simulink model "GridS"  (R2022a)
settings: Solver=FixedStepDiscrete  StartTime=0.0  StopTime=5  RelTol=1e-3
values from neighbouring files (symbols this model uses):
  Clink = Ceq*2    (= 0.217013888889)    [Set_parameters_R2018.m]
  Fc = 33 * Fnom    (= 1980)    [Set_parameters_R2018.m]
  Fnom = 60    [Set_parameters_R2018.m]
  Increment_MPPT = 0.01    [Set_parameters_R2018.m]
  Ki_Ireg = 20    [Set_parameters_R2018.m]
  Ki_VDCreg = 400    [Set_parameters_R2018.m]
  Kp_Ireg = 0.3    [Set_parameters_R2018.m]
  Kp_VDCreg = 2    [Set_parameters_R2018.m]
  LimitL_Ireg = -1.5    [Set_parameters_R2018.m]
  LimitL_VDCreg = -1.5    [Set_parameters_R2018.m]
  Limits_MPPT = [ 583 357 ]    [Set_parameters_R2018.m]
  LimitU_Ireg = 1.5    [Set_parameters_R2018.m]
  LimitU_VDCreg = 1.5    [Set_parameters_R2018.m]
  Pnom = 1e6    (= 1000000)    [Set_parameters_R2018.m]
  Ts_Control = 10*Ts_Power    (= 5.05050505051e-05)    [Set_parameters_R2018.m]
  Ts_Power = 1/(33*Fnom)/100    (= 5.05050505051e-06)    [Set_parameters_R2018.m]
  Vf = 0    [Set_parameters_R2018.m]
  Vfd = 0    [Set_parameters_R2018.m]
  Vnom_dc = 480    [Set_parameters_R2018.m]
  Vnom_Diesel = 2.4e3    (= 2400)    [Set_parameters_R2018.m]
  Vnom_prim = 13.8e3    (= 13800)    [Set_parameters_R2018.m]
  Vnom_sec = 220    [Set_parameters_R2018.m]
undefined symbols (not defined in the file or in its folder): D1, Delta, RL, RLff, sigbuilder_block
libraries: spsLoadFlowBusLib x7, spsThreePhasePISectionLineLib x6, spsThreePhaseSeriesRLCLoadLib x4, spsThreePhaseTransformerTwoWindingsLib x3, spsThreePhaseBreakerLib x2, spsThreePhaseVIMeasurementLib x2, spsThreePhaseSeriesRLCBranchLib x2, spsSeriesRLCBranchLib x2, slpidlib x2, spsabctodq0Lib x2, spsVoltageMeasurementLib x2, spsPVArrayLib x1
settings Model: Creator=z0034ktr  LastModifiedBy=pdutt
settings SolverCC: AlgebraicLoopSolver=TrustRegion
settings DebuggingCC: IgnoredZcDiagnostic=none  UnconnectedInputMsg=warning  UnconnectedOutputMsg=warning  UnconnectedLineMsg=warning  SFMachineParentedDataDiag=warning

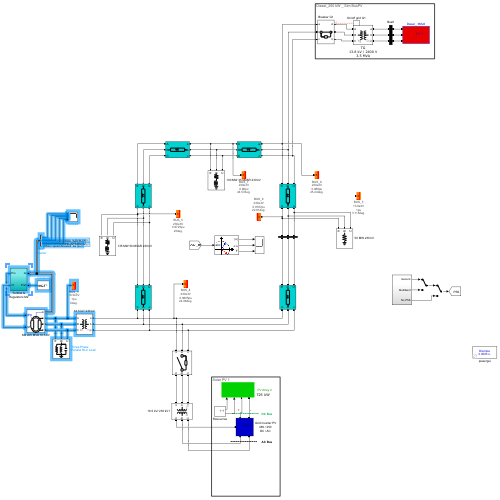
[thumbnail: Simulink's stored preview of the top-level diagram]
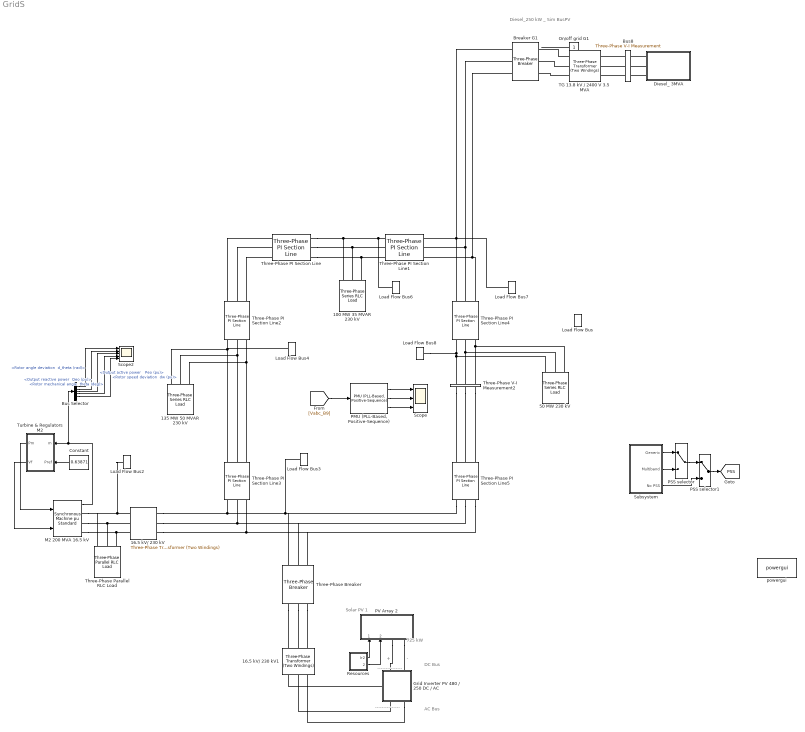
== system GridS ==
  note: -
  note: +
  note: ---------------
  note: ---------------
  note: Solar PV 1
  note: 725 kW
  note: DC Bus
  note: AC Bus
  note: Diesel_250 kW _ Sim BusPV
  "  PV Array 2" : Subsystem
      mask Display: image(imread('Icons\PV.png'));
  100 MW 35 MVAR 230 kV : spsThreePhaseSeriesRLCLoadLib/Three-Phase Series RLC Load  LConnTagsString=A|B|C  Configuration=Y (grounded)  NominalVoltage=(230000)*0.980041  Vabc=[1e3 1e3 1e3]  Vabcp=[1e3 1e3 1e3]  NominalFrequency=60  UnbalancedPower=off  ActivePower=100e6  InductivePower=35e6  CapacitivePower=0  Pabc=[10e3 9e3 11e3]  QLabc=[100 90 110]  QCabc=[100 90 110]  Pabcp=[10e3 9e3 11e3]  QLabcp=[100 90 110]  QCabcp=[100 90 110]  Measurements=None  LoadType=constant PQ
  135 MW 50 MVAR 230 kV : spsThreePhaseSeriesRLCLoadLib/Three-Phase Series RLC Load  LConnTagsString=A|B|C  Configuration=Y (grounded)  NominalVoltage=(230000)*0.972469  Vabc=[1e3 1e3 1e3]  Vabcp=[1e3 1e3 1e3]  NominalFrequency=60  UnbalancedPower=off  ActivePower=135e6  InductivePower=50e6  CapacitivePower=0  Pabc=[10e3 9e3 11e3]  QLabc=[100 90 110]  QCabc=[100 90 110]  Pabcp=[10e3 9e3 11e3]  QLabcp=[100 90 110]  QCabcp=[100 90 110]  Measurements=None  LoadType=constant PQ
  16.5 kV/ 230 kV : spsThreePhaseTransformerTwoWindingsLib/Three-Phase Transformer (Two Windings)  Winding1Connection=Delta (D1)  Winding2Connection=Yg  CoreType=Three single-phase transformers  SetSaturation=off  Hysteresis=off  DataFile='hysteresis'  SetInitialFlux=off  Measurements=None  UNITS=pu  NominalPower=[ 200e6 , 60 ]  Winding1=[ 16.5e3 , 0.002 , 0.08 ]  Winding2=[ 230e3 , 0.002 , 0.08 ]  Rm=500  Lm=500  L0=0.5  Saturation=[ 0,0 ; 0.0024,1.2 ; 1.0,1.52 ]  InitialFluxes=[ 0.8 , -0.8 , 0.7 ]  BreakLoop=off  DiscreteSolver=Trapezoidal iterative  DataType=off  TransfoNumber=1
  16.5 kV/ 230 kV1 : spsThreePhaseTransformerTwoWindingsLib/Three-Phase Transformer (Two Windings)  Winding1Connection=Delta (D1)  Winding2Connection=Yg  CoreType=Three single-phase transformers  SetSaturation=off  Hysteresis=off  DataFile='hysteresis'  SetInitialFlux=off  Measurements=None  UNITS=pu  NominalPower=[ 200e6 , 60 ]  Winding1=[ 250 , 0.002 , 0.08 ]  Winding2=[ 230e3 , 0.002 , 0.08 ]  Rm=500  Lm=500  L0=0.5  Saturation=[ 0,0 ; 0.0024,1.2 ; 1.0,1.52 ]  InitialFluxes=[ 0.8 , -0.8 , 0.7 ]  BreakLoop=off  DiscreteSolver=Trapezoidal iterative  DataType=off  TransfoNumber=1
  50 MW 230 kV : spsThreePhaseSeriesRLCLoadLib/Three-Phase Series RLC Load  LConnTagsString=A|B|C  Configuration=Y (grounded)  NominalVoltage=(230000)*0.978663  Vabc=[1e3 1e3 1e3]  Vabcp=[1e3 1e3 1e3]  NominalFrequency=60  UnbalancedPower=off  ActivePower=50e6  InductivePower=0  CapacitivePower=0  Pabc=[10e3 9e3 11e3]  QLabc=[100 90 110]  QCabc=[100 90 110]  Pabcp=[10e3 9e3 11e3]  QLabcp=[100 90 110]  QCabcp=[100 90 110]  Measurements=None  LoadType=constant PQ
  Breaker G1 : spsThreePhaseBreakerLib/Three-Phase Breaker  InitialState=closed  SwitchA=on  SwitchB=on  SwitchC=on  SwitchTimes=[3 5]  External=off  BreakerResistance=0.001  SnubberResistance=1e6  SnubberCapacitance=inf  Measurements=None
  Bus Selector : BusSelector  OutputSignals="Mechanical.Rotor angle deviation  d_theta (rad),Output reactive power  Qeo (pu),Output active power   Peo (pu),Mechanical.Rotor mechanical angle  theta (deg),Mechanical.Rotor speed deviation  dw (pu)"
  Bus8 : spsThreePhaseVIMeasurementLib/Three-Phase V-I Measurement  VoltageMeasurement=phase-to-ground  SetLabelV=on  LabelV=VabcLL_Bus_8  Vpu=off  VpuLL=off  CurrentMeasurement=yes  SetLabelI=on  LabelI=IabcLL_Bus_8  Ipu=off  Pbase=100e6  Vbase=25e3/sqrt(2)  OutputType=Complex  PhasorSimulation=off  PSBequivalent=0
  Constant : Constant  Value=0.63871
  Diesel_ 3MVA : Subsystem
      mask Display: image(imread('Icons\Diesel 50kW1.png'));
  "Grid Inverter PV 480 / 250 DC / AC " : Subsystem
      settings: PortSchema="{\"entries\":[{\"content\":{\"sides\":[{\"content\":{\"connectorIds\":[\"LConn1\",\"LConn2\"]},\"type\":\"ConnectorPlacement.EquallySpacedRectSide\",\"uuid\":\"ac79584a-c7d0-4a74-aa4d-67aed92924e2\"},{\"content\":{\"connectorIds\":[\"RConn1\",\"RConn2\"],\"side\":\"RIGHT\"},\"type\":\"ConnectorPlacement.EquallySpacedRectSide\",\"uuid\":\"44d96f25-a8f9-47e8-b296-82c7ffbfe922\"},{\"content\":{\"connectorIds\":[\"LConn3\"],\"side\":\"TOP\"},\"type\":\"ConnectorPlacement.EquallySpacedRectSide\",\"uuid\":\"f35e0256-66c3-4b52-94e0-36412c815474\"}]},\"type\":\"ConnectorPlacement.EquallySpacedConnector\",\"uuid\":\"6af4db4f-53ba-4d1f-a030-0edda350e303\"}],\"packageUris\":[\"http://schema.mathworks.com/mf0/Connector/R2020b\"],\"version\":\"1.0\"}"
      mask Display: image(imread('Icons\Inverter.png'));
  Load Flow Bus : spsLoadFlowBusLib/Load Flow Bus  LConnTagsString=a  Phases=single  Connectors=on one side  ID=BUS_3  Vbase=13.8e3  Vref=1  Vangle=0  VLF=1  VLFb=1  VLFc=1  angleLF=3.115  angleLFb=0  angleLFc=0
      settings: SourceProductBaseCode=PS
  Load Flow Bus2 : spsLoadFlowBusLib/Load Flow Bus  LConnTagsString=a  Phases=single  Connectors=on one side  ID=BUS_1  Vbase=16.5e3  Vref=1  Vangle=0  VLF=1  VLFb=1  VLFc=1  angleLF=0  angleLFb=0  angleLFc=0
      settings: SourceProductBaseCode=PS
  Load Flow Bus3 : spsLoadFlowBusLib/Load Flow Bus  LConnTagsString=a  Phases=single  Connectors=on one side  ID=BUS_4  Vbase=230e3  Vref=1  Vangle=0  VLF=0.9805  VLFb=1  VLFc=1  angleLF=24.06  angleLFb=0  angleLFc=0
      settings: SourceProductBaseCode=PS
  Load Flow Bus4 : spsLoadFlowBusLib/Load Flow Bus  LConnTagsString=a  Phases=single  Connectors=on one side  ID=BUS_5  Vbase=230e3  Vref=1  Vangle=0  VLF=0.9725  VLFb=1  VLFc=1  angleLF=23  angleLFb=0  angleLFc=0
      settings: SourceProductBaseCode=PS
  Load Flow Bus6 : spsLoadFlowBusLib/Load Flow Bus  LConnTagsString=a  Phases=single  Connectors=on one side  ID=BUS_7  Vbase=230e3  Vref=1  Vangle=0  VLF=0.98  VLFb=1  VLFc=1  angleLF=24.57  angleLFb=0  angleLFc=0
      settings: SourceProductBaseCode=PS
  Load Flow Bus7 : spsLoadFlowBusLib/Load Flow Bus  LConnTagsString=a  Phases=single  Connectors=on one side  ID=BUS_8  Vbase=230e3  Vref=1  Vangle=0  VLF=0.988  VLFb=1  VLFc=1  angleLF=25.24  angleLFb=0  angleLFc=0
      settings: SourceProductBaseCode=PS
  Load Flow Bus8 : spsLoadFlowBusLib/Load Flow Bus  LConnTagsString=a  Phases=single  Connectors=on one side  ID=BUS_9  Vbase=230e3  Vref=1  Vangle=0  VLF=0.9787  VLFb=1  VLFc=1  angleLF=22.61  angleLFb=0  angleLFc=0
      settings: SourceProductBaseCode=PS
  M2 200 MVA 16.5 kV : spsSynchronousMachinepuStandardLib/Synchronous Machine pu Standard  PresetModel=No  MechanicalLoad=Mechanical power Pm  ShowDetailedParameters=on  RotorType=Salient-pole  Units=per unit standard parameters  MeasurementBus=off  NominalParameters="[200E6  16500   60 ]"  Reactances1=[ 31 32 33 34 35 36 37 ]  Reactances2=[ 1.305, 0.296, 0.252, 0.474, 0.243, 0.18 ]  dAxisTimeConstants=Short-circuit  qAxisTimeConstants=Open-circuit  TimeConstants1=[]  TimeConstants2=[]  TimeConstants3=[]  TimeConstants4=[]  TimeConstants5=[ 1.01, 0.053, 0.1 ]  TimeConstants6=[]  TimeConstants7=[]  TimeConstants8=[]  StatorResistance=2.8544e-3  Mechanical="[ 3.7 0  32]"  PolePairs=32  InitialConditions=[0 -74.1936 0.653801 0.653801 0.653801 -12.3345 -132.335 107.665 1.36624]  SetSaturation=off  Saturation=[0.6404,0.7127,0.8441,0.9214,0.9956,1.082,1.19,1.316,1.457;0.7,0.7698,0.8872,0.9466,0.9969,1.046,1.1,1.151,1.201]  LoadFlowParameters=[2 4000000000 0 0]  TsPowergui=0  TsBlock=-1  IterativeModel=Trapezoidal non iterative  IterativeDiscreteModel=Trapezoidal non iterative  BusType=swing  Pref=0  Qref=0  Qmin=-Inf  Qmax=Inf  PLF=0  QLF=0
      settings: SourceProductName=Specialized Power Systems
  On/off grid G1 : Constant
  "PMU (PLL-Based, Positive-Sequence)" : spsPMUPLLBasedPositiveSequenceLib/PMU (PLL-Based, Positive-Sequence)  nominalFrequency=60  samplingRate=64  reportingFactor=1
      settings: SourceProductBaseCode=PS
  PSS selector : ManualSwitch
  PSS selector1 : ManualSwitch
  Resources : Subsystem
      mask Display: image(imread('Icons\R_Sol.jpg'));
  Scope : Scope  NumInputPorts=3
  Scope2 : Scope  NumInputPorts=5
  Subsystem : Subsystem
  TG 13.8 kV / 2400 V 3.5 MVA : spsThreePhaseTransformerTwoWindingsLib/Three-Phase Transformer (Two Windings)  Winding1Connection=Yg  Winding2Connection=Delta (D1)  CoreType=Three single-phase transformers  SetSaturation=off  Hysteresis=off  DataFile='hysteresis'  SetInitialFlux=off  Measurements=None  UNITS=pu  NominalPower=[3.5e6 , Fnom ]  Winding1=[ 230e3, 0.015/2 , 0.015/2/377]  Winding2=[ Vnom_Diesel , 0.015/2 , 0.015/2/377]  Rm=500  Lm=500  L0=0.5  Saturation="[ 0,0  ;  0.005,1.2  ;  1.0,1.4 ]"  InitialFluxes=[ 0.8 , -0.8 , 0.7 ]  BreakLoop=off  DiscreteSolver=Trapezoidal iterative  DataType=off  TransfoNumber=0
  Three-Phase PI Section Line : spsThreePhasePISectionLineLib/Three-Phase PI Section Line  LConnTagsString=a|b|c  RConnTagsString=A|B|C  Length=50  Frequency=60  Resistances=[ 0.01273 0.3864]  Inductances="[ 0.9337e-3  4.1264e-3]"  Capacitances=[12.74e-9 7.751e-9]
  Three-Phase PI Section Line1 : spsThreePhasePISectionLineLib/Three-Phase PI Section Line  LConnTagsString=a|b|c  RConnTagsString=A|B|C  Length=100  Frequency=60  Resistances=[ 0.01273 0.3864]  Inductances="[ 0.9337e-3  4.1264e-3]"  Capacitances=[12.74e-9 7.751e-9]
  Three-Phase PI Section Line2 : spsThreePhasePISectionLineLib/Three-Phase PI Section Line  LConnTagsString=a|b|c  RConnTagsString=A|B|C  Length=100  Frequency=60  Resistances=[ 0.01273 0.3864]  Inductances="[ 0.9337e-3  4.1264e-3]"  Capacitances=[12.74e-9 7.751e-9]
  Three-Phase PI Section Line3 : spsThreePhasePISectionLineLib/Three-Phase PI Section Line  LConnTagsString=a|b|c  RConnTagsString=A|B|C  Length=50  Frequency=60  Resistances=[ 0.01273 0.3864]  Inductances="[ 0.9337e-3  4.1264e-3]"  Capacitances=[12.74e-9 7.751e-9]
  Three-Phase PI Section Line4 : spsThreePhasePISectionLineLib/Three-Phase PI Section Line  LConnTagsString=a|b|c  RConnTagsString=A|B|C  Length=100  Frequency=60  Resistances=[ 0.01273 0.3864]  Inductances="[ 0.9337e-3  4.1264e-3]"  Capacitances=[12.74e-9 7.751e-9]
  Three-Phase PI Section Line5 : spsThreePhasePISectionLineLib/Three-Phase PI Section Line  LConnTagsString=a|b|c  RConnTagsString=A|B|C  Length=50  Frequency=60  Resistances=[ 0.01273 0.3864]  Inductances="[ 0.9337e-3  4.1264e-3]"  Capacitances=[12.74e-9 7.751e-9]
  Three-Phase Parallel RLC Load : spsThreePhaseParallelRLCLoadLib/Three-Phase Parallel RLC Load  LConnTagsString=A|B|C  Configuration=Y (grounded)  NominalVoltage=16.5e3  Vabc=[1e3 1e3 1e3]  Vabcp=[1e3 1e3 1e3]  NominalFrequency=60  UnbalancedPower=off  ActivePower=10e3  InductivePower=100  CapacitivePower=100  Pabc=[10e3 9e3 11e3]  QLabc=[100 90 110]  QCabc=[100 90 110]  Pabcp=[10e3 9e3 11e3]  QLabcp=[100 90 110]  QCabcp=[100 90 110]  Measurements=None  LoadType=constant Z
  Three-Phase V-I Measurement2 : spsThreePhaseVIMeasurementLib/Three-Phase V-I Measurement  VoltageMeasurement=phase-to-phase  SetLabelV=on  LabelV=Vabc_B9  Vpu=off  VpuLL=on  CurrentMeasurement=no  SetLabelI=off  LabelI=Iabc  Ipu=off  Pbase=100e6  Vbase=230e3  OutputType=Complex  PhasorSimulation=off  PSBequivalent=0
  Three-Phase Breaker : spsThreePhaseBreakerLib/Three-Phase Breaker  InitialState=open  SwitchA=on  SwitchB=on  SwitchC=on  SwitchTimes=[2 5]  External=off  BreakerResistance=0.01  SnubberResistance=1e6  SnubberCapacitance=inf  Measurements=None
  Turbine & Regulators M2 : Subsystem
  powergui : spspowerguiLib/powergui  Priority=1  SimulationMode=Discrete  SampleTime=50e-5  frequency=60  Iterations=50  frequencyindice=60  Pbase=200  ErrMax=0.0001  UnitsV=kV  UnitsW=MW  buscounter=0  FunctionMessages=off  echomessages=off  EnableUseOfTLC=off  CurrentSourceSwitches=off  DisableSnubberDevices=off  DisableRonSwitches=off  DisableVfSwitches=off  DisplayEquations=off  AutomaticDiscreteSolvers=off  SolverType=Backward Euler  Interpol=off  ExternalGateDelay=off  methode=off  Ts=100  x0status=blocks  SPID=on  SwTol=0  HookPort=off  NonlinearTolerance=1e-4  nMaxIteration=100  ContinueOnMaxIteration=off  RestoreLinks=warning  ResistiveCurrentMeasurement=off  Frange=[0:2:500]  Ylog=off  Xlog=on  ShowGrid=off  save=off  variable=ZData  structure=0  ZoomFFT=off  StartTime=0.0  cycles=1  DisplayStyle=1  fundamental=60  FreqAxis=off  MaxFrequency=1000  frequencyindicesteady=1  RmsSteady=1  display=off
  tag scope: PSS=global
  wires:
  [Vabc_B9] -> "PMU (PLL-Based, Positive-Sequence)"/1
  "PMU (PLL-Based, Positive-Sequence)"/3 -> Scope/3
  "PMU (PLL-Based, Positive-Sequence)"/2 -> Scope/2
  "PMU (PLL-Based, Positive-Sequence)"/1 -> Scope/1
  M2 200 MVA 16.5 kV/1 -> Bus Selector/1, Turbine & Regulators M2/1(m)
  Turbine & Regulators M2/2(Vf) -> M2 200 MVA 16.5 kV/2
  Turbine & Regulators M2/1(Pm) -> M2 200 MVA 16.5 kV/1
  Constant/1 -> Turbine & Regulators M2/2(Pref)
  PSS selector/1 -> PSS selector1/1
  Subsystem/1(Generic) -> PSS selector/1
  Subsystem/3(No PSS) -> PSS selector1/2
  Subsystem/2(Multiband) -> PSS selector/2
  PSS selector1/1 -> [PSS]
  Bus Selector/1 -> Scope2/1  "<Rotor angle deviation  d_theta (rad)>"
  Bus Selector/2 -> Scope2/2  "<Output reactive power  Qeo (pu)>"
  Bus Selector/3 -> Scope2/3  "<Output active power   Peo (pu)>"
  Bus Selector/4 -> Scope2/4  "<Rotor mechanical angle  theta (deg)>"
  Bus Selector/5 -> Scope2/5  "<Rotor speed deviation  dw (pu)>"
  Resources/1(Ir2) -> "  PV Array 2"/1(Irradiance)
  Resources/2(temp) -> "  PV Array 2"/2(Temp2)
  On/off grid G1/1 -> ?
  connections:
  16.5 kV/ 230 kV/RConn1 -- Three-Phase Breaker/RConn1 -- Three-Phase PI Section Line5/RConn1 -- Load Flow Bus3/LConn1 -- Three-Phase PI Section Line3/RConn1
  16.5 kV/ 230 kV/RConn2 -- Three-Phase Breaker/RConn2 -- Three-Phase PI Section Line5/RConn2 -- Three-Phase PI Section Line3/RConn2
  16.5 kV/ 230 kV/RConn3 -- Three-Phase Breaker/RConn3 -- Three-Phase PI Section Line5/RConn3 -- Three-Phase PI Section Line3/RConn3
  50 MW 230 kV/LConn1 -- Three-Phase PI Section Line4/RConn1 -- Load Flow Bus8/LConn1 -- Three-Phase V-I Measurement2/RConn1
  Three-Phase V-I Measurement2/LConn3 -- Three-Phase PI Section Line5/LConn3
  Three-Phase PI Section Line4/LConn1 -- Breaker G1/RConn1 -- Load Flow Bus7/LConn1 -- Three-Phase PI Section Line1/RConn1
  Three-Phase PI Section Line4/LConn2 -- Breaker G1/RConn2 -- Three-Phase PI Section Line1/RConn2
  Three-Phase PI Section Line4/LConn3 -- Breaker G1/RConn3 -- Three-Phase PI Section Line1/RConn3
  Three-Phase PI Section Line/RConn1 -- 100 MW 35 MVAR 230 kV/LConn1 -- Load Flow Bus6/LConn1 -- Three-Phase PI Section Line1/LConn1
  Three-Phase PI Section Line/RConn2 -- 100 MW 35 MVAR 230 kV/LConn2 -- Three-Phase PI Section Line1/LConn2
  Three-Phase PI Section Line/RConn3 -- 100 MW 35 MVAR 230 kV/LConn3 -- Three-Phase PI Section Line1/LConn3
  Three-Phase PI Section Line3/LConn1 -- Load Flow Bus4/LConn1 -- Three-Phase PI Section Line2/RConn1 -- 135 MW 50 MVAR 230 kV/LConn1
  Three-Phase PI Section Line3/LConn2 -- 135 MW 50 MVAR 230 kV/LConn2 -- Three-Phase PI Section Line2/RConn2
  Three-Phase PI Section Line3/LConn3 -- 135 MW 50 MVAR 230 kV/LConn3 -- Three-Phase PI Section Line2/RConn3
  Three-Phase PI Section Line2/LConn3 -- Three-Phase PI Section Line/LConn3
  Three-Phase PI Section Line2/LConn2 -- Three-Phase PI Section Line/LConn2
  Three-Phase PI Section Line2/LConn1 -- Three-Phase PI Section Line/LConn1
  Load Flow Bus2/LConn1 -- Three-Phase Parallel RLC Load/LConn1 -- M2 200 MVA 16.5 kV/RConn1 -- 16.5 kV/ 230 kV/LConn1
  M2 200 MVA 16.5 kV/RConn2 -- 16.5 kV/ 230 kV/LConn2 -- Three-Phase Parallel RLC Load/LConn2
  M2 200 MVA 16.5 kV/RConn3 -- 16.5 kV/ 230 kV/LConn3 -- Three-Phase Parallel RLC Load/LConn3
  50 MW 230 kV/LConn3 -- Three-Phase V-I Measurement2/RConn3 -- Three-Phase PI Section Line4/RConn3
  Three-Phase V-I Measurement2/LConn2 -- Three-Phase PI Section Line5/LConn2
  Three-Phase V-I Measurement2/LConn1 -- Three-Phase PI Section Line5/LConn1
  50 MW 230 kV/LConn2 -- Three-Phase V-I Measurement2/RConn2 -- Three-Phase PI Section Line4/RConn2
  "  PV Array 2"/LConn1 -- "Grid Inverter PV 480 / 250 DC / AC "/LConn1
  "  PV Array 2"/LConn2 -- "Grid Inverter PV 480 / 250 DC / AC "/LConn2
  "Grid Inverter PV 480 / 250 DC / AC "/LConn3 -- 16.5 kV/ 230 kV1/LConn1
  "Grid Inverter PV 480 / 250 DC / AC "/RConn1 -- 16.5 kV/ 230 kV1/LConn2
  "Grid Inverter PV 480 / 250 DC / AC "/RConn2 -- 16.5 kV/ 230 kV1/LConn3
  Three-Phase Breaker/LConn1 -- 16.5 kV/ 230 kV1/RConn1
  Three-Phase Breaker/LConn2 -- 16.5 kV/ 230 kV1/RConn2
  Three-Phase Breaker/LConn3 -- 16.5 kV/ 230 kV1/RConn3
  Bus8/RConn3 -- TG 13.8 kV / 2400 V 3.5 MVA/RConn3
  Diesel_ 3MVA/LConn1 -- Bus8/LConn1
  Diesel_ 3MVA/LConn2 -- Bus8/LConn2
  TG 13.8 kV / 2400 V 3.5 MVA/LConn2 -- Breaker G1/LConn2
  Bus8/RConn1 -- TG 13.8 kV / 2400 V 3.5 MVA/RConn1
  TG 13.8 kV / 2400 V 3.5 MVA/LConn3 -- Breaker G1/LConn3
  TG 13.8 kV / 2400 V 3.5 MVA/LConn1 -- Breaker G1/LConn1
  Bus8/RConn2 -- TG 13.8 kV / 2400 V 3.5 MVA/RConn2
  Diesel_ 3MVA/LConn3 -- Bus8/LConn3

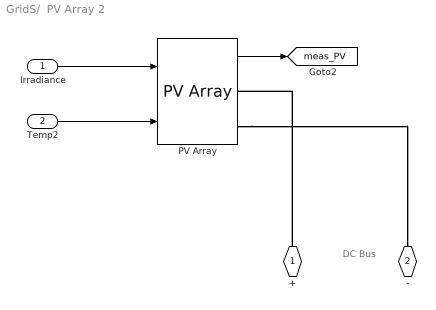
== system GridS/  PV Array 2 ==
  note: DC Bus
  Irradiance : Inport
  Temp2 : Inport  Port=2
  PV Array : spsPVArrayLib/PV Array  Npar=250  Nser=7  PlotType=array @ 1000 W/m2 & specified temperatures  S_vec="[ 1000  500  100 ]"  Temp_C_vec="[ 45 25  ]"  ModuleName=SunPower SPR-415E-WHT-D  PlotWhenSelected=off  Pm=414.801  Ncell=128  Voc=85.3  Isc=6.09  Vm=72.9  Im=5.69  beta_Voc_pc=-0.229  alpha_Isc_pc=0.030706  beta_Voc=-0.19534  alpha_Isc=0.00187  IL=6.0978  I0=7.1698e-13  nI=0.87223  Rsh=419.7781  Rs=0.53711  RobustModel=off  RobustCellTemperature=313.3991  BAL=on  Tc=1e-6  Tfilter=5e-5
      settings: AttributesFormatString=|
      | %<ModuleName>
      | %<Nser>-module string
      | %<Npar> parallel strings
  + : PMIOPort  Tag=PMCPort  Side=Left
  - : PMIOPort  Tag=PMCPort  Port=2  Side=Left
  tag scope: meas_PV=global
  wires:
  PV Array/1 -> [meas_PV]
  Irradiance/1 -> PV Array/1
  Temp2/1 -> PV Array/2
  connections:
  PV Array/RConn2 -- -/RConn1
  +/RConn1 -- PV Array/RConn1

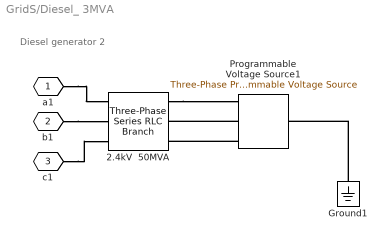
== system GridS/Diesel_ 3MVA ==
  note: Diesel generator 2
  2.4kV  50MVA : spsThreePhaseSeriesRLCBranchLib/Three-Phase Series RLC Branch  LConnTagsString=A|B|C  RConnTagsString=A|B|C  BranchType=RL  Resistance=2.4e3^2/50e6/10  Inductance=2.4e3^2/50e6/(2*pi*60)  Capacitance=1.0  Measurements=None
  Ground1 : spsGroundLib/Ground  LConnTagsString=a
  Programmable Voltage Source1 : spsThreePhaseProgrammableVoltageSourceLib/Three-Phase Programmable Voltage Source  PositiveSequence="[Vnom_Diesel*0.9848 -60  Fnom]"  VariationEntity=None  VariationType=Table of time-amplitude pairs  VariationTypeAlt=Step  VariationStep=-0.3  VariationRate=0.5  VariationMagnitude=0.4  VariationFrequency=2  VariationTiming=[0.1 1.2]  VariationPhaseA=off  Amplitudes=[1]  TimeValues=[0]  HarmonicGeneration=off  HarmonicA=[3 0.2 -25 0]  HarmonicB="[2 0.15  35 2]"  Timing="[0.1  0.6]"  BusType=PV  Pref=Pgen_Diesel  Qref=0  Qmin=-inf  Qmax=inf
  a1 : PMIOPort  Tag=PMCPort  Side=Left
  b1 : PMIOPort  Tag=PMCPort  Port=2  Side=Left
  c1 : PMIOPort  Tag=PMCPort  Port=3  Side=Left
  connections:
  Programmable Voltage Source1/RConn3 -- 2.4kV  50MVA/LConn3
  Ground1/LConn1 -- Programmable Voltage Source1/LConn1
  Programmable Voltage Source1/RConn2 -- 2.4kV  50MVA/LConn2
  2.4kV  50MVA/LConn1 -- Programmable Voltage Source1/RConn1
  b1/RConn1 -- 2.4kV  50MVA/RConn2
  a1/RConn1 -- 2.4kV  50MVA/RConn1
  c1/RConn1 -- 2.4kV  50MVA/RConn3

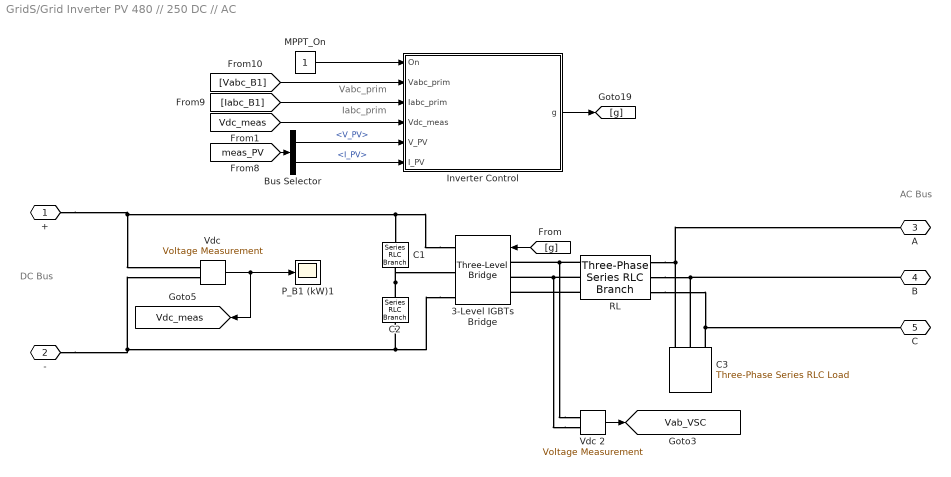
== system GridS/Grid Inverter PV 480 // 250 DC // AC  ==
  note: Iabc_prim
  note: Vabc_prim
  note: AC Bus
  note: DC Bus
  3-Level IGBTs Bridge : spsThreeLevelBridgeLib/Three-Level Bridge  Arms=3  SnubberResistance=Rs  SbubberCapacitance=Cs  Device=IGBT / Diodes  Ron=Ron  ForwardVoltages="[  Vfd  Vf ]"  Measurements=None
      settings: AttributesFormatString=\n  SourceProductBaseCode=PS
  Bus Selector : BusSelector  OutputSignals=V_PV,I_PV
  C1 : spsSeriesRLCBranchLib/Series RLC Branch  LConnTagsString=__new0  RConnTagsString=__new0  BranchType=C  Resistance=1.0  Inductance=1.0  SetiL0=off  InitialCurrent=0  Capacitance=Clink  Setx0=on  InitialVoltage=Vnom_dc/2  Measurements=None
  C2 : spsSeriesRLCBranchLib/Series RLC Branch  LConnTagsString=__new0  RConnTagsString=__new0  BranchType=C  Resistance=1.0  Inductance=1.0  SetiL0=off  InitialCurrent=0  Capacitance=Clink  Setx0=on  InitialVoltage=Vnom_dc/2  Measurements=None
  C3 : spsThreePhaseSeriesRLCLoadLib/Three-Phase Series RLC Load  LConnTagsString=A|B|C  Configuration=Delta  NominalVoltage=Vnom_sec  Vabc=[1e3 1e3 1e3]  Vabcp=[1e3 1e3 1e3]  NominalFrequency=Fnom  UnbalancedPower=off  ActivePower=Pc  InductivePower=0  CapacitivePower=Qc  Pabc=[10e3 9e3 11e3]  QLabc=[100 90 110]  QCabc=[100 90 110]  Pabcp=[10e3 9e3 11e3]  QLabcp=[100 90 110]  QCabcp=[100 90 110]  Measurements=None  LoadType=constant Z
  Inverter Control : Subsystem  mask(Inverter Control){Pnom=Pnom, Fnom=Fnom, Vnom_prim=Vnom_prim, Vnom_sec=Vnom_sec, Vnom_dc=Vnom_dc, Increment_MPPT=Increment_MPPT, Limits_MPPT=Limits_MPPT, Vdc_ref_Init=Vnom_dc, Kp_VDCreg=Kp_VDCreg, Ki_VDCreg=Ki_VDCreg, Kp_Ireg=Kp_Ireg, Ki_Ireg=Ki_Ireg, RLff=RLff, Fc=Fc, Ts_Control=Ts_Control, Ts_PWMgenerator=Ts_Power}
      mask prompts: Pnom "Power (VA)"; Fnom "Frequency (Hz)"; Vnom_prim "Primary voltage (Vrms LL)"; Vnom_sec "Secondary voltage (Vrms LL)"; Vnom_dc "DC voltage (V)"; Increment_MPPT "Output increment (V)"; Limits_MPPT "Output limits [ Upper  Lower ]"; Vdc_ref_Init "Output initial value (V)"; Kp_VDCreg "Proportional gain"; Ki_VDCreg "Integral gain"; Kp_Ireg "Proportional gain"; Ki_Ireg "Integral gain"; RLff "Feedforward Values [Rff Lff]"; Fc "Carrier frequency (Hz)"; Ts_Control "Control systems"; Ts_PWMgenerator "PWM generator"
      mask help:
      | The main components of the Inverter Control are:
      | 1. PLL & Measurements
      | 2. Maximum Power Point Tracker System (MPPT) using a Perturb & Observe algorithm
      | 3. DC Voltage Regulator
      | 4. Current Regulator
      | 5. PWM Modulator
      mask DialogControl Container4 Prompt: Nominal Values:
      mask DialogControl Container3 Prompt: MPPT Controller:
      mask DialogControl Container8 Prompt: Dc Voltage Regulator:
      mask DialogControl Container6 Prompt: Current Regulator:
      mask DialogControl Container9 Prompt: PWM Modulator:
      mask DialogControl SampleTimes Prompt: Sample Times:
      mask Display: image('Icons\FPGA.png');
  MPPT_On : Constant
  P_B1 (kW)1 : Scope
  RL : spsThreePhaseSeriesRLCBranchLib/Three-Phase Series RLC Branch  LConnTagsString=A|B|C  RConnTagsString=A|B|C  BranchType=RL  Resistance=RL(1)  Inductance=RL(2)  Capacitance=inf  Measurements=None
  "Vdc " : spsVoltageMeasurementLib/Voltage Measurement  Tag=PoWeRsYsTeMmEaSuReMeNt  PhasorSimulation=off  OutputType=Magnitude  PSBequivalent=0
  Vdc 2 : spsVoltageMeasurementLib/Voltage Measurement  Tag=PoWeRsYsTeMmEaSuReMeNt  PhasorSimulation=off  OutputType=Magnitude  PSBequivalent=0
  + : PMIOPort  Side=Left
  - : PMIOPort  Port=2  Side=Left
  A : PMIOPort  Port=3  Side=Left
  B : PMIOPort  Port=4  Side=Right
  C : PMIOPort  Port=5  Side=Right
  tag scope: Vab_VSC=global, Vdc_meas=global
  wires:
  Bus Selector/1 -> Inverter Control/5(V_PV)  "<V_PV>"
  [Vdc_meas] -> Inverter Control/4(Vdc_meas)
  [meas_PV] -> Bus Selector/1
  MPPT_On/1 -> Inverter Control/1(On)
  [Vabc_B1] -> Inverter Control/2(Vabc_prim)
  [Iabc_B1] -> Inverter Control/3(Iabc_prim)
  Bus Selector/2 -> Inverter Control/6(I_PV)  "<I_PV>"
  "Vdc "/1 -> [Vdc_meas], P_B1 (kW)1/1
  Vdc 2/1 -> [Vab_VSC]
  Inverter Control/1(g) -> [g]
  [g] -> 3-Level IGBTs Bridge/1
  connections:
  Vdc 2/LConn1 -- 3-Level IGBTs Bridge/LConn1 -- RL/LConn1
  Vdc 2/LConn2 -- 3-Level IGBTs Bridge/LConn2 -- RL/LConn2
  C3/LConn1 -- RL/RConn1 -- A/RConn1
  C3/LConn2 -- RL/RConn2 -- B/RConn1
  3-Level IGBTs Bridge/RConn3 -- -/RConn1 -- "Vdc "/LConn2 -- C2/RConn1
  C1/RConn1 -- C2/LConn1 -- 3-Level IGBTs Bridge/RConn2
  3-Level IGBTs Bridge/RConn1 -- C1/LConn1 -- "Vdc "/LConn1 -- +/RConn1
  RL/LConn3 -- 3-Level IGBTs Bridge/LConn3
  C3/LConn3 -- RL/RConn3 -- C/RConn1

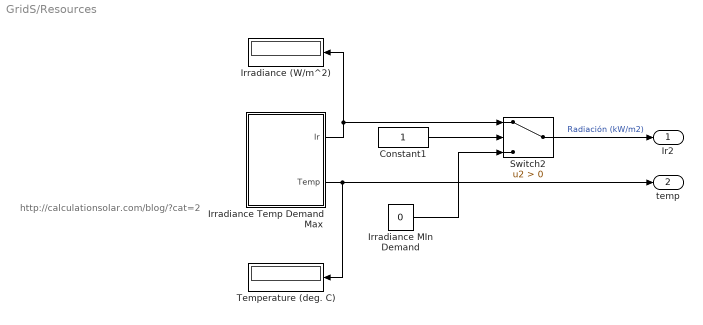
== system GridS/Resources ==
  note: http://calculationsolar.com/blog/?cat=2
  Constant1 : Constant
  Irradiance (W/m^2) : Display
      settings: Format=bank  Decimation=1000
  Irradiance Temp Demand Max : Subsystem  Tag=STV Subsys  LoadFcn=sigbuilder_block('load');  StartFcn=sigbuilder_block('start');  StopFcn=sigbuilder_block('stop');  ClipboardFcn=sigbuilder_block('clipboard');  mask(Sigbuilder block){tuvar=[0:10]}
      mask help: Sigbuilder GUI
      mask init:
      | if ~strcmp(get_param(bdroot(gcbh),'SimulationStatus'),'stopped') tuvar = sigbuilder_block('maskInit'); end
      settings: CopyFcn=sigbuilder_block('copy');  DeleteFcn=sigbuilder_block('delete');  ModelCloseFcn=sigbuilder_block('modelClose');  PreSaveFcn=sigbuilder_block('preSave');  PauseFcn=sigbuilder_block('pause')  ContinueFcn=sigbuilder_block('continue')  NameChangeFcn=sigbuilder_block('namechange');  OpenFcn=sigbuilder_block('open',[0 30 1024.5 488.25 ]);  CloseFcn=sigbuilder_block('close');
      mask Display: plot(0, 0, 100, 100,[2, 2, 32, 32, 2], [68, 8, 8, 68, 68],[32, 2], [38, 38], [32, 19, 2],[53, 60, 44], [32, 17, 17, 2],[16, 16, 31, 31]);txt = getActiveGroup(gcbh);text(2, 100, txt,'verticalAlignment', 'top');
  Irradiance MIn Demand : Constant  Value=0
  Switch2 : Switch  Criteria=u2 > Threshold  SaturateOnIntegerOverflow=off  InputSameDT=off
  Temperature (deg. C) : Display
      settings: Format=bank  Decimation=1000
  Ir2 : Outport  VectorParamsAs1DForOutWhenUnconnected=off
  temp : Outport  Port=2  VectorParamsAs1DForOutWhenUnconnected=off
  wires:
  Constant1/1 -> Switch2/2
  Irradiance Temp Demand Max/2(Temp) -> temp/1, Temperature (deg. C)/1
  Irradiance MIn Demand/1 -> Switch2/3
  Switch2/1 -> Ir2/1  "Radiación (kW/m2)"
  Irradiance Temp Demand Max/1(Ir) -> Switch2/1, Irradiance (W/m^2)/1

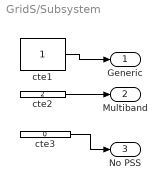
== system GridS/Subsystem ==
  cte1 : Constant
  cte2 : Constant  Value=2
  cte3 : Constant  Value=0
  Generic : Outport  VectorParamsAs1DForOutWhenUnconnected=off
  Multiband : Outport  Port=2  VectorParamsAs1DForOutWhenUnconnected=off
  No PSS : Outport  Port=3  VectorParamsAs1DForOutWhenUnconnected=off
  wires:
  cte1/1 -> Generic/1
  cte2/1 -> Multiband/1
  cte3/1 -> No PSS/1

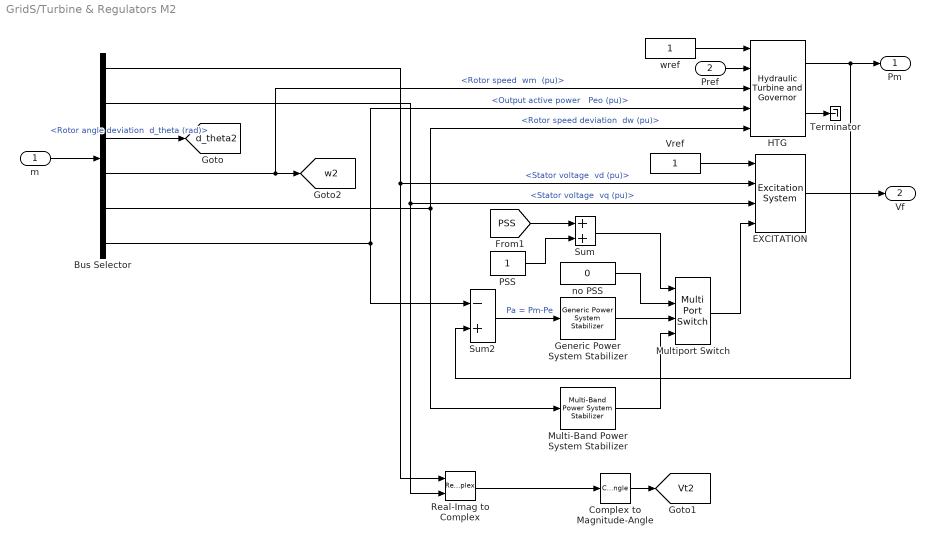
== system GridS/Turbine & Regulators M2 ==
  m : Inport
  Pref : Inport  Port=2
  Bus Selector : BusSelector  OutputSignals="dq0 components.Stator voltage  vd (pu),dq0 components.Stator voltage  vq (pu),Mechanical.Rotor angle deviation  d_theta (rad),Mechanical.Rotor speed  wm  (pu),Mechanical.Rotor speed deviation  dw (pu),Output active power   Peo (pu)"
  Complex to Magnitude-Angle : ComplexToMagnitudeAngle  Output=Magnitude
  EXCITATION : spsExcitationSystemLib/Excitation System  tr=20e-3  reg=[ 200, 0.001 ]  exc=[ 1, 0 ]  tgr=[ 0, 0 ]  damp=[ 0.001, 0.1 ]  sat=[ 0, 0 ]  lim="[ 0,  7, 0 ]"  v0=[1 1.3662]
      settings: SourceProductName=Specialized Power Systems
  Generic Power System Stabilizer : spsGenericPowerSystemStabilizerLib/Generic Power System Stabilizer  Tsensor=15e-3  K=2  Twashout=0.7  Tleadlag1="[60e-3  0.5]"  Tleadlag2=[0 0]  VSlimits=[-0.15 0.15]  Vinit=0  Plot_On=off  MagdB_On=on  FreqRange=logspace(-2,2,500)
      settings: SourceProductName=Specialized Power Systems
  HTG : spsHydraulicTurbineandGovernorLib/Hydraulic Turbine and Governor  sm="[ 10/3  0.07 ]"  gate="[  0.01  0.97518  -0.1  0.1 ]"  reg="[  0.05  1.163  0.105  0  0.01  ]"  hyd="[  0  2.67  ]"  dref=0  po=0.63993
      settings: SourceProductName=Specialized Power Systems
  Multi-Band Power System Stabilizer : spsMultiBandPowerSystemStabilizerLib/Multi-Band Power System Stabilizer  OperationMode=Simplified settings  Kg=1.0  GL=[0.025 5]  GI=[0.8 25]  GH=[12.0 145]  GLd=[66 66 9.4]  TcLF=[1.667 2 0 0 0 0 2 2.4 0 0 0 0 1 1]  GId=[66 66 47.6]  TcIF=[1 1 0.25 0.3 0 0 1 1 0.3 0.36 0 0 0 0]  GHd=[66 66 233]  TcHF="[0.01 0.012 0 0 0 0  0.012 0.0144 0 0 0 0 1 1]"  LIM=[.075 .15 .15 .15]  Plot_On=off  MagdB_On=off  FreqRange=logspace(-2,2,500)
      settings: SourceProductName=Specialized Power Systems
  Multiport Switch : MultiPortSwitch  InputSameDT=off
  PSS : Constant
  Real-Imag to Complex : RealImagToComplex
  Sum : Sum  SaturateOnIntegerOverflow=on
  Sum2 : Sum  Inputs=-+  InputSameDT=on  SaturateOnIntegerOverflow=on  OutDataTypeStr=Inherit: Same as first input
  Terminator : Terminator
  Vref : Constant
  no PSS : Constant  Value=0
  wref : Constant
  Pm : Outport  InitialOutput=0  VectorParamsAs1DForOutWhenUnconnected=off
  Vf : Outport  Port=2  InitialOutput=0  VectorParamsAs1DForOutWhenUnconnected=off
  tag scope: Vt2=global, d_theta2=global, w2=global
  wires:
  PSS/1 -> Sum/2
  [PSS] -> Sum/1
  Real-Imag to Complex/1 -> Complex to Magnitude-Angle/1
  HTG/2 -> Terminator/1
  Vref/1 -> EXCITATION/1
  m/1 -> Bus Selector/1
  Bus Selector/5 -> HTG/5, Multi-Band Power System Stabilizer/1  "<Rotor speed deviation  dw (pu)>"
  Bus Selector/6 -> Sum2/1, HTG/4  "<Output active power   Peo (pu)>"
  Bus Selector/4 -> [w2], HTG/3  "<Rotor speed  wm  (pu)>"
  Pref/1 -> HTG/2
  wref/1 -> HTG/1
  HTG/1 -> Pm/1, Sum2/2
  Bus Selector/2 -> Real-Imag to Complex/2, EXCITATION/3  "<Stator voltage  vq (pu)>"
  EXCITATION/1 -> Vf/1
  Bus Selector/1 -> Real-Imag to Complex/1, EXCITATION/2  "<Stator voltage  vd (pu)>"
  Complex to Magnitude-Angle/1 -> [Vt2]
  Bus Selector/3 -> [d_theta2]  "<Rotor angle deviation  d_theta (rad)>"
  Sum2/1 -> Generic Power System Stabilizer/1  "Pa = Pm-Pe"
  Generic Power System Stabilizer/1 -> Multiport Switch/3
  Multi-Band Power System Stabilizer/1 -> Multiport Switch/4
  no PSS/1 -> Multiport Switch/2
  Sum/1 -> Multiport Switch/1
  Multiport Switch/1 -> EXCITATION/4

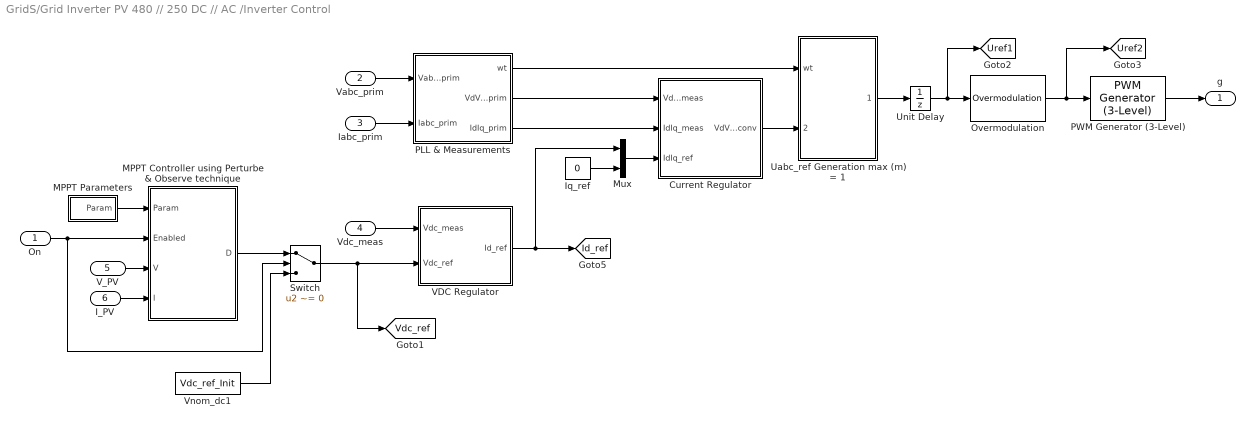
== system GridS/Grid Inverter PV 480 // 250 DC // AC /Inverter Control ==
  On : Inport  PortDimensions=1
  Vabc_prim : Inport  Port=2  PortDimensions=3
  Iabc_prim : Inport  Port=3  PortDimensions=3
  Vdc_meas : Inport  Port=4  PortDimensions=1
  V_PV : Inport  Port=5  PortDimensions=1
  I_PV : Inport  Port=6  PortDimensions=1
  Current Regulator : Subsystem
  Iq_ref : Constant  Value=0
  MPPT Parameters : Subsystem
  "MPPT Controller using Perturbe & Observe technique " : MATLAB Function  TreatAsAtomicUnit=on
  Mux : Mux  Inputs=2
  Overmodulation : spsOvermodulationLib/Overmodulation  OverModType=Flat top
      settings: SourceProductBaseCode=PS
  PLL & Measurements : Subsystem
  PWM Generator (3-Level) : spsPWMGenerator3LevelLib/PWM Generator (3-Level)  ModulatorType=Three-phase bridge (12 pulses)  ModulatorMode=Unsynchronized  nF=27  Fc=Fc  ModulatingSignals=off  m=0.8  Freq=60  Phase=0  Ts=Ts_PWMgenerator
      settings: SourceProductBaseCode=PS
  Switch : Switch  Criteria=u2 ~= 0  SaturateOnIntegerOverflow=off  InputSameDT=off
  Uabc_ref Generation max (m) = 1 : Subsystem
  Unit Delay : UnitDelay  SampleTime=Ts_Control  HasFrameUpgradeWarning=on
  VDC Regulator : Subsystem
  Vnom_dc1 : Constant  Value=Vdc_ref_Init
  g : Outport  VectorParamsAs1DForOutWhenUnconnected=off
  tag scope: Id_ref=global, Uref1=global, Uref2=global, Vdc_ref=global
  wires:
  PLL & Measurements/1(wt) -> Uabc_ref Generation max (m) = 1/1(wt)
  Current Regulator/1(VdVq_conv) -> Uabc_ref Generation max (m) = 1/2(VdVq_conv)
  Iq_ref/1 -> Mux/2
  Mux/1 -> Current Regulator/3(IdIq_ref)
  PLL & Measurements/3(IdIq_prim) -> Current Regulator/2(IdIq_meas)
  PLL & Measurements/2(VdVq_prim) -> Current Regulator/1(VdVq_meas)
  Vabc_prim/1 -> PLL & Measurements/1(Vabc_prim)
  Iabc_prim/1 -> PLL & Measurements/2(Iabc_prim)
  PWM Generator (3-Level)/1 -> g/1
  Vdc_meas/1 -> VDC Regulator/1(Vdc_meas)
  VDC Regulator/1(Id_ref) -> [Id_ref], Mux/1
  V_PV/1 -> "MPPT Controller using Perturbe & Observe technique "/3(V)
  I_PV/1 -> "MPPT Controller using Perturbe & Observe technique "/4(I)
  MPPT Parameters/1(Param) -> "MPPT Controller using Perturbe & Observe technique "/1(Param)
  On/1 -> "MPPT Controller using Perturbe & Observe technique "/2(Enabled), Switch/2
  Overmodulation/1 -> [Uref2], PWM Generator (3-Level)/1
  Unit Delay/1 -> [Uref1], Overmodulation/1
  "MPPT Controller using Perturbe & Observe technique "/1(D) -> Switch/1
  Switch/1 -> [Vdc_ref], VDC Regulator/2(Vdc_ref)
  Vnom_dc1/1 -> Switch/3
  Uabc_ref Generation max (m) = 1/1(Uabc_ref) -> Unit Delay/1

== system GridS/Resources/Irradiance Temp Demand Max ==
  Demux : Demux  Tag=STV Demux  Outputs=2
      settings: DisplayOption=none
  FromWs : FromWorkspace  Tag=STV FromWs  VariableName=tuvar
      SigBuilderData=|
      | common.afterFinalStr = 'Extrapolate'
      | common.sampleTime = '0'
      | dataSet(1).timeRange = [0 2]
      | dataSet(1).name = 'Constant Irradiance'
      | dataSet(2).timeRange = [0 2]
      | dataSet(2).name = 'Step Irradiance'
      | dataSet(3).timeRange = [0 3]
      | dataSet(3).name = 'Ramp-up/down Irradiance'
      | sbobj.Groups(1).Name = 'Constant Irradiance'
      | sbobj.Groups(1).Signals(1).Name = 'Ir'
      | sbobj.Groups(1).Signals(1).XData = [0 2]
      | sbobj.Groups(1).Signals(1).YData = [1000 1000]
      | sbobj.Groups(1).Signals(2).Name = 'Temp'
      | sbobj.Groups(1).Signals(2).XData = [0 1 1 2]
      | sbobj.Groups(1).Signals(2).YData = [0 0 1 1]
      | sbobj.Groups(1).TimeRange = [0 2]
      | sbobj.Groups(2).Name = 'Step Irradiance'
      | sbobj.Groups(2).Signals(1).Name = 'Ir'
      | sbobj.Groups(2).Signals(1).XData = [0 0.252 0.252 2]
      | sbobj.Groups(2).Signals(1).YData = [600 600 1000 1000]
      | sbobj.Groups(2).Signals(2).Name = 'Temp'
      | sbobj.Groups(2).Signals(2).XData = [0 1 1 2]
      | sbobj.Groups(2).Signals(2).YData = [0 0 1 1]
      | sbobj.Groups(2).TimeRange = [0 2]
      | sbobj.Groups(3).Name = 'Ramp-up/down Irradiance'
      | sbobj.Groups(3).Signals(1).Name = 'Ir'
      | sbobj.Groups(3).Signals(1).XData = [0 0.785 1.7 2.28 3]
      | sbobj.Groups(3).Signals(1).YData = [1000 999.538235294 999 999.446153846 1000]
      | sbobj.Groups(3).Signals(2).Name = 'Temp'
      | sbobj.Groups(3).Signals(2).XData = [0 2 2.1 3]
      | sbobj.Groups(3).Signals(2).YData = [25 25 25 25]
      | sbobj.Groups(3).TimeRange = [0 3]
  Ir : Outport  Tag=STV Outport  VectorParamsAs1DForOutWhenUnconnected=off
  Temp : Outport  Tag=STV Outport  Port=2  VectorParamsAs1DForOutWhenUnconnected=off
  wires:
  Demux/1 -> Ir/1
  FromWs/1 -> Demux/1
  Demux/2 -> Temp/1

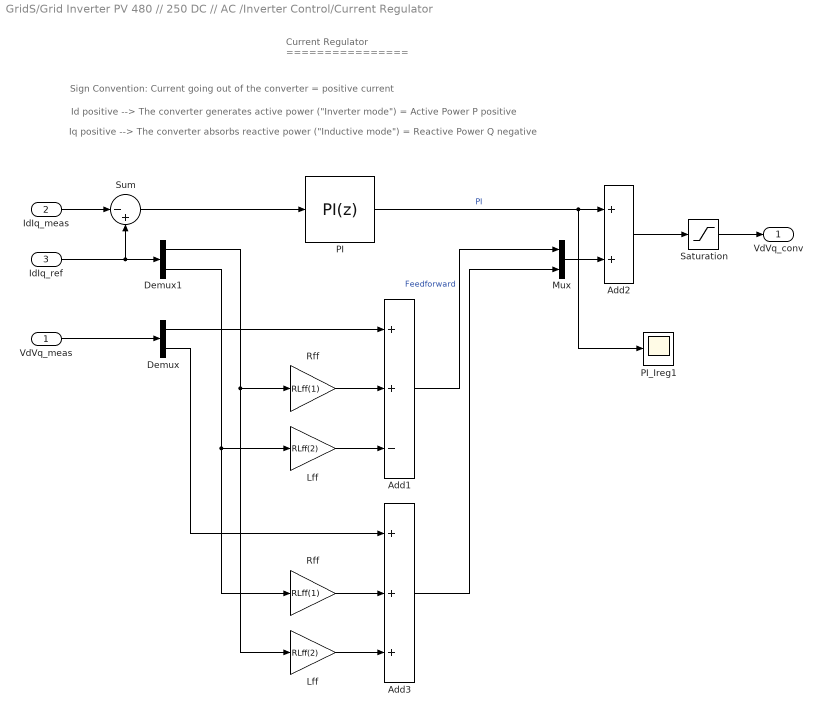
== system GridS/Grid Inverter PV 480 // 250 DC // AC /Inverter Control/Current Regulator ==
  note: Current Regulator
      | ================
  note: Sign Convention: Current going out of the converter = positive current
  note: Iq positive --> The converter absorbs reactive power ("Inductive mode") = Reactive Power Q negative
  note: Id positive --> The converter generates active power ("Inverter mode") = Active Power P positive
  VdVq_meas : Inport  PortDimensions=2
  IdIq_meas : Inport  Port=2  PortDimensions=2
  IdIq_ref : Inport  Port=3  PortDimensions=2
  Add1 : Sum  Inputs=++-
  Add2 : Sum
  Add3 : Sum  Inputs=+++
  Demux : Demux  Outputs=2
  Demux1 : Demux  Outputs=2
  Lff : Gain  Gain=RLff(2)  SaturateOnIntegerOverflow=on  OutDataTypeStr=Inherit: Same as input  ParamDataTypeStr=Inherit: Same as input
  "Lff  " : Gain  Gain=RLff(2)  SaturateOnIntegerOverflow=on  OutDataTypeStr=Inherit: Same as input  ParamDataTypeStr=Inherit: Same as input
  Mux : Mux  Inputs=2
  PI : slpidlib/PID Controller  Controller=PI  Form=Parallel  TimeDomain=Discrete-time  UseExternalTs=off  SampleTime=Ts_Control  IntegratorMethod=Forward Euler  FilterMethod=Forward Euler  ControllerParametersSource=internal  P=Kp_Ireg  I=Ki_Ireg  UseKiTs=off  D=0  N=100  UseFilter=on  TunerSelectOption=Transfer Function Based (PID Tuner App)  InitialConditionSource=internal  InitialConditionForIntegrator=0  InitialConditionForFilter=0  DifferentiatorICPrevScaledInput=0  ExternalReset=none  TrackingMode=off  Kt=1  LimitOutput=on  SatLimitsSource=internal  UpperSaturationLimit=LimitU_Ireg  LowerSaturationLimit=LimitL_Ireg  LinearizeAsGain=off  AntiWindupMode=none  Kb=1  POutMin=[]  POutMax=[]  IOutMin=[]  IOutMax=[]  DOutMin=[]  DOutMax=[]  NOutMin=[]  NOutMax=[]  SumOutMin=[]  SumOutMax=[]  SaturationOutMin=[]  SaturationOutMax=[]  PParamMin=[]  PParamMax=[]  IParamMin=[]  IParamMax=[]  DParamMin=[]  DParamMax=[]  NParamMin=[]  NParamMax=[]  KbParamMin=[]  KbParamMax=[]  KtParamMin=[]  KtParamMax=[]  KbOutMin=[]  KbOutMax=[]  KtOutMin=[]  KtOutMax=[]  IntegratorOutMin=[]  IntegratorOutMax=[]  FilterOutMin=[]  FilterOutMax=[]  SumI1OutMin=[]  SumI1OutMax=[]  SumI2OutMin=[]  SumI2OutMax=[]  SumI3OutMin=[]  SumI3OutMax=[]  SumI4OutMin=[]  SumI4OutMax=[]  SumDOutMin=[]  SumDOutMax=[]  DifferentiatorOutMin=[]  DifferentiatorOutMax=[]  FilterDiffOutCoefMin=[]  FilterDiffOutCoefMax=[]  ReciprocalOutMin=[]  ReciprocalOutMax=[]  SumDenOutMin=[]  SumDenOutMax=[]  SumNumOutMin=[]  SumNumOutMax=[]  DivideOutMin=[]  DivideOutMax=[]  UdiffTsProdOutMin=[]  UdiffTsProdOutMax=[]  NTsProdOutMin=[]  NTsProdOutMax=[]  UintegralTsProdOutMin=[]  UintegralTsProdOutMax=[]  UngainTsProdOutMin=[]  UngainTsProdOutMax=[]  IntegratorContinuousStateAttributes=''  IntegratorStateMustResolveToSignalObject=off  IntegratorRTWStateStorageClass=Auto  FilterContinuousStateAttributes=''  FilterStateMustResolveToSignalObject=off  FilterRTWStateStorageClass=Auto  ParallelPVariant=InternalParameters  IdealPVariant=Disabled  IVariant=InternalParameters  DVariant=Disabled  IntegratorVariant=Discrete  SatVariant=Enabled  AWVariant=Passthrough  PCopyVariant=Disabled  TRVariant=Disabled  FdbkBlocksVariant=Forward  IdealPFdbkVariant=Disabled  SatFdbkVariant=Disabled  DerivativeFilterVariant=Disabled  NVariant=Disabled  NCopyVariant=Disabled_SignalSpec  FilterICVariant=Disabled  IntegratorICVariant=InternalICs  ExternalResetVariant=Disabled  TRSumVariant=Passthrough  SumFdbkVariant=Disabled  SumVariant=Sum_PI  TsampFilterVariant=InternalTs  TsampNgainVariant=Passthrough  TsampIntegralVariant=Passthrough  ExternalSaturationOutDataTypeStr=Inherit: Same as second input  aMode=0
  PI_Ireg1 : Scope
  Rff : Gain  Gain=RLff(1)  SaturateOnIntegerOverflow=on  OutDataTypeStr=Inherit: Same as input  ParamDataTypeStr=Inherit: Same as input
  "Rff " : Gain  Gain=RLff(1)  SaturateOnIntegerOverflow=on  OutDataTypeStr=Inherit: Same as input  ParamDataTypeStr=Inherit: Same as input
  Saturation : Saturate  UpperLimit=LimitU_Ireg  LowerLimit=LimitL_Ireg
  Sum : Sum  Inputs=|-+
  VdVq_conv : Outport  VectorParamsAs1DForOutWhenUnconnected=off
  wires:
  Mux/1 -> Add2/2
  PI/1 -> PI_Ireg1/1, Add2/1  "PI"
  Sum/1 -> PI/1
  IdIq_ref/1 -> Sum/2, Demux1/1
  IdIq_meas/1 -> Sum/1
  Add2/1 -> Saturation/1
  Saturation/1 -> VdVq_conv/1
  VdVq_meas/1 -> Demux/1
  Demux/1 -> Add1/1
  "Rff "/1 -> Add1/2
  Demux1/1 -> "Rff "/1, Lff/1
  "Lff  "/1 -> Add1/3
  Demux1/2 -> "Lff  "/1, Rff/1
  Rff/1 -> Add3/2
  Lff/1 -> Add3/3
  Add1/1 -> Mux/1  "Feedforward"
  Demux/2 -> Add3/1
  Add3/1 -> Mux/2

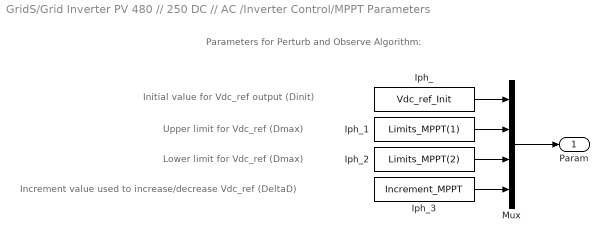
== system GridS/Grid Inverter PV 480 // 250 DC // AC /Inverter Control/MPPT Parameters ==
  note: Parameters for Perturb and Observe Algorithm:
  note: Lower limit for Vdc_ref (Dmax)
  note: Initial value for Vdc_ref output (Dinit)
  note: Increment value used to increase/decrease Vdc_ref (DeltaD)
  note: Upper limit for Vdc_ref (Dmax)
  Iph_ : Constant  Value=Vdc_ref_Init
  Iph_1 : Constant  Value=Limits_MPPT(1)
  Iph_2 : Constant  Value=Limits_MPPT(2)
  Iph_3 : Constant  Value=Increment_MPPT
  Mux : Mux
  Param : Outport  VectorParamsAs1DForOutWhenUnconnected=off
  wires:
  Mux/1 -> Param/1
  Iph_3/1 -> Mux/4
  Iph_2/1 -> Mux/3
  Iph_1/1 -> Mux/2
  Iph_/1 -> Mux/1

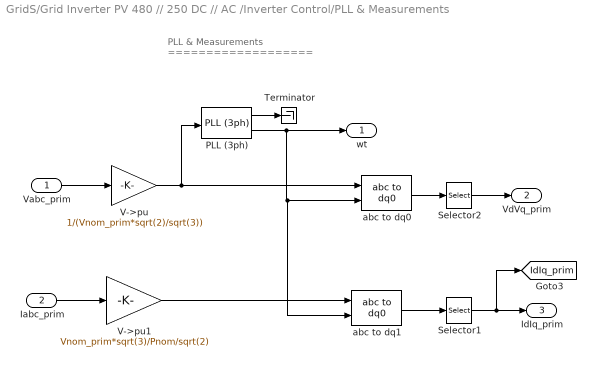
== system GridS/Grid Inverter PV 480 // 250 DC // AC /Inverter Control/PLL & Measurements ==
  note: PLL & Measurements
      | ===================
  Vabc_prim : Inport
  Iabc_prim : Inport  Port=2
  PLL (3ph) : spsPLL3phLib/PLL (3ph)  Fmin=45  Par_Init="[-0.57  Fnom]"  ParK=[180, 3200, 1]  TcD=1e-4  MaxRateChangeFreq=12  FilterCutOffFreq=25  Ts=Ts_Control  AGC=on
  Selector1 : Selector  InputPortWidth=3  IndexOptions=Index vector (dialog)  Indices=[1 2]  OutputSizes=1
  Selector2 : Selector  InputPortWidth=3  IndexOptions=Index vector (dialog)  Indices=[1 2]  OutputSizes=1
  Terminator : Terminator
  V->pu : Gain  Gain=1/(Vnom_prim*sqrt(2)/sqrt(3))  SaturateOnIntegerOverflow=on  OutDataTypeStr=Inherit: Same as input  ParamDataTypeStr=Inherit: Same as input
  V->pu1 : Gain  Gain=Vnom_prim*sqrt(3)/Pnom/sqrt(2)  SaturateOnIntegerOverflow=on  OutDataTypeStr=Inherit: Same as input  ParamDataTypeStr=Inherit: Same as input
  abc to dq0 : spsabctodq0Lib/abc to dq0  Alignment=90 degrees behind phase A axis
  abc to dq1 : spsabctodq0Lib/abc to dq0  Alignment=90 degrees behind phase A axis
  wt : Outport  VectorParamsAs1DForOutWhenUnconnected=off
  VdVq_prim : Outport  Port=2  VectorParamsAs1DForOutWhenUnconnected=off
  IdIq_prim : Outport  Port=3  VectorParamsAs1DForOutWhenUnconnected=off
  tag scope: IdIq_prim=global
  wires:
  V->pu1/1 -> abc to dq1/1
  V->pu/1 -> PLL (3ph)/1, abc to dq0/1
  abc to dq1/1 -> Selector1/1
  Vabc_prim/1 -> V->pu/1
  Iabc_prim/1 -> V->pu1/1
  abc to dq0/1 -> Selector2/1
  Selector2/1 -> VdVq_prim/1
  Selector1/1 -> [IdIq_prim], IdIq_prim/1
  PLL (3ph)/2 -> wt/1, abc to dq1/2, abc to dq0/2
  PLL (3ph)/1 -> Terminator/1

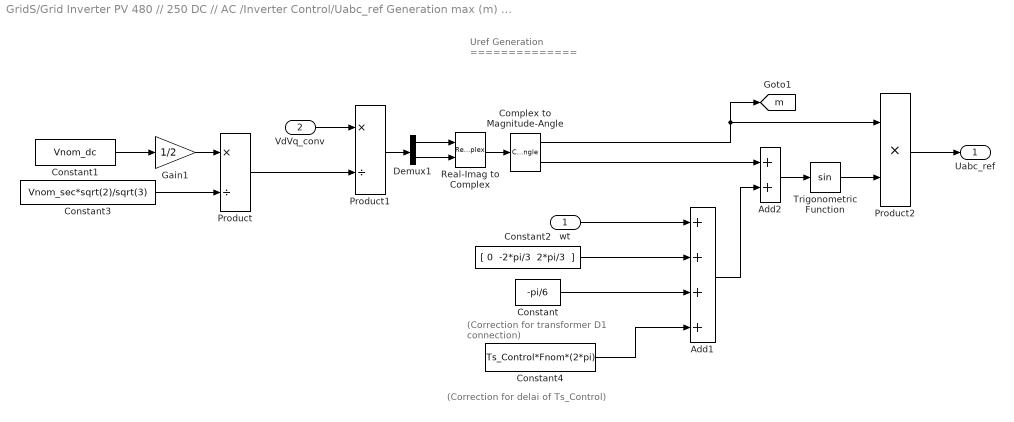
== system GridS/Grid Inverter PV 480 // 250 DC // AC /Inverter Control/Uabc_ref Generation max (m) = 1 ==
  note: (Correction for transformer
      |  D1 connection)
  note: (Correction for delai of Ts_Control)
  note: Uref Generation
      | ==============
  wt : Inport
  VdVq_conv : Inport  Port=2
  Add1 : Sum  Inputs=++++
  Add2 : Sum
  Complex to Magnitude-Angle : ComplexToMagnitudeAngle
  Constant : Constant  Value=-pi/6
  Constant1 : Constant  Value=Vnom_dc
  Constant2 : Constant  Value="[ 0  -2*pi/3  2*pi/3  ]"
  Constant3 : Constant  Value=Vnom_sec*sqrt(2)/sqrt(3)
  Constant4 : Constant  Value=Ts_Control*Fnom*(2*pi)
  Demux1 : Demux  Outputs=2
  Gain1 : Gain  Gain=1/2
  Product : Product  Inputs=*/  RndMeth=Zero
  Product1 : Product  Inputs=*/  RndMeth=Zero
  Product2 : Product  Inputs=**  RndMeth=Zero
  Real-Imag to Complex : RealImagToComplex
  Trigonometric Function : Trigonometry
  Uabc_ref : Outport  VectorParamsAs1DForOutWhenUnconnected=off
  tag scope: m=global
  wires:
  Constant1/1 -> Gain1/1
  VdVq_conv/1 -> Product1/1
  Product1/1 -> Demux1/1
  Gain1/1 -> Product/1
  Real-Imag to Complex/1 -> Complex to Magnitude-Angle/1
  Demux1/1 -> Real-Imag to Complex/1
  Demux1/2 -> Real-Imag to Complex/2
  Constant2/1 -> Add1/2
  Constant/1 -> Add1/3
  Constant3/1 -> Product/2
  Product/1 -> Product1/2
  Complex to Magnitude-Angle/2 -> Add2/1
  Add1/1 -> Add2/2
  Add2/1 -> Trigonometric Function/1
  Complex to Magnitude-Angle/1 -> [m], Product2/1
  Trigonometric Function/1 -> Product2/2
  Product2/1 -> Uabc_ref/1
  wt/1 -> Add1/1
  Constant4/1 -> Add1/4

== system GridS/Grid Inverter PV 480 // 250 DC // AC /Inverter Control/VDC Regulator ==
  Vdc_meas : Inport  PortDimensions=1
  Vdc_ref : Inport  Port=2  PortDimensions=1
  PI : slpidlib/PID Controller  Controller=PI  Form=Parallel  TimeDomain=Discrete-time  UseExternalTs=off  SampleTime=Ts_Control  IntegratorMethod=Trapezoidal  FilterMethod=Forward Euler  ControllerParametersSource=internal  P=Kp_VDCreg  I=Ki_VDCreg  UseKiTs=off  D=0  N=100  UseFilter=on  TunerSelectOption=Transfer Function Based (PID Tuner App)  InitialConditionSource=internal  InitialConditionForIntegrator=1  InitialConditionForFilter=0  DifferentiatorICPrevScaledInput=0  ExternalReset=none  TrackingMode=off  Kt=1  LimitOutput=on  SatLimitsSource=internal  UpperSaturationLimit=LimitU_VDCreg  LowerSaturationLimit=LimitL_VDCreg  LinearizeAsGain=off  AntiWindupMode=none  Kb=1  POutMin=[]  POutMax=[]  IOutMin=[]  IOutMax=[]  DOutMin=[]  DOutMax=[]  NOutMin=[]  NOutMax=[]  SumOutMin=[]  SumOutMax=[]  SaturationOutMin=[]  SaturationOutMax=[]  PParamMin=[]  PParamMax=[]  IParamMin=[]  IParamMax=[]  DParamMin=[]  DParamMax=[]  NParamMin=[]  NParamMax=[]  KbParamMin=[]  KbParamMax=[]  KtParamMin=[]  KtParamMax=[]  KbOutMin=[]  KbOutMax=[]  KtOutMin=[]  KtOutMax=[]  IntegratorOutMin=[]  IntegratorOutMax=[]  FilterOutMin=[]  FilterOutMax=[]  SumI1OutMin=[]  SumI1OutMax=[]  SumI2OutMin=[]  SumI2OutMax=[]  SumI3OutMin=[]  SumI3OutMax=[]  SumI4OutMin=[]  SumI4OutMax=[]  SumDOutMin=[]  SumDOutMax=[]  DifferentiatorOutMin=[]  DifferentiatorOutMax=[]  FilterDiffOutCoefMin=[]  FilterDiffOutCoefMax=[]  ReciprocalOutMin=[]  ReciprocalOutMax=[]  SumDenOutMin=[]  SumDenOutMax=[]  SumNumOutMin=[]  SumNumOutMax=[]  DivideOutMin=[]  DivideOutMax=[]  UdiffTsProdOutMin=[]  UdiffTsProdOutMax=[]  NTsProdOutMin=[]  NTsProdOutMax=[]  UintegralTsProdOutMin=[]  UintegralTsProdOutMax=[]  UngainTsProdOutMin=[]  UngainTsProdOutMax=[]  IntegratorContinuousStateAttributes=''  IntegratorStateMustResolveToSignalObject=off  IntegratorRTWStateStorageClass=Auto  FilterContinuousStateAttributes=''  FilterStateMustResolveToSignalObject=off  FilterRTWStateStorageClass=Auto  ParallelPVariant=InternalParameters  IdealPVariant=Disabled  IVariant=InternalParameters  DVariant=Disabled  IntegratorVariant=Discrete  SatVariant=Enabled  AWVariant=Passthrough  PCopyVariant=Disabled  TRVariant=Disabled  FdbkBlocksVariant=Forward  IdealPFdbkVariant=Disabled  SatFdbkVariant=Disabled  DerivativeFilterVariant=Disabled  NVariant=Disabled  NCopyVariant=Disabled_SignalSpec  FilterICVariant=Disabled  IntegratorICVariant=InternalICs  ExternalResetVariant=Disabled  TRSumVariant=Passthrough  SumFdbkVariant=Disabled  SumVariant=Sum_PI  TsampFilterVariant=InternalTs  TsampNgainVariant=Passthrough  TsampIntegralVariant=Passthrough  ExternalSaturationOutDataTypeStr=Inherit: Same as second input  aMode=0
  Rtot_pu3 : Gain  Gain=1/Vnom_dc  SaturateOnIntegerOverflow=on  OutDataTypeStr=Inherit: Same as input  ParamDataTypeStr=Inherit: Same as input
  Sum : Sum  Inputs=|+-
  Id_ref : Outport  InitialOutput=0  VectorParamsAs1DForOutWhenUnconnected=off
  wires:
  PI/1 -> Id_ref/1
  Rtot_pu3/1 -> PI/1
  Vdc_ref/1 -> Sum/2
  Vdc_meas/1 -> Sum/1
  Sum/1 -> Rtot_pu3/1

== matlab function GridS/Grid Inverter PV 480 // 250 DC // AC /Inverter Control/MPPT Controller using Perturbe & Observe technique  ==
  settings: updateMethod=DISCRETE  sampleTime=Ts_Control
  data: Param input; Enabled input; V input =V; I input; D output
function D  = PandO(Param, Enabled, V, I)

% MPPT controller based on the Perturb & Observe algorithm.

% D output = Reference for DC link voltage (Vdc_ref) 
%
% Enabled input = 1 to enable the MPPT controller
% V input = PV array terminal voltage (V)
% I input = PV array current (A)
%
% Param input:
Dinit = Param(1);  %Initial value for Vdc_ref
Dmax = Param(2);   %Maximum value for Vdc_ref
Dmin = Param(3);   %Minimum value for Vdc_ref
deltaD = Param(4); %Increment value used to increase/decrease Vdc_ref
%  

persistent Vold Pold Dold;

dataType = 'double';

if isempty(Vold)
    Vold=0;
    Pold=0;
    Dold=Dinit;
end
P= V*I;
dV= V - Vold;
dP= P - Pold;

if dP ~= 0 & Enabled ~=0
    if dP < 0
        if dV < 0
            D = Dold + deltaD;
        else
            D = Dold - deltaD;
        end
    else
        if dV < 0
            D = Dold - deltaD;
        else
            D = Dold + deltaD;
        end    
    end
else D=Dold;
end

if D >= Dmax | D<= Dmin
    D=Dold;
end

Dold=D;
Vold=V;
Pold=P;
